simulink model "NL_Simulation"  (R2018b)
settings: Solver=VariableStepAuto  StartTime=0.0  StopTime=.5  FixedStep=0.01
values from neighbouring files (symbols this model uses):
  StateVals = SetInitial(Vinf,AeroType)    [setup_NL.m]
undefined symbols (not defined in the file or in its folder): AC
libraries: Tools_6dofSimulation x12, aerolibatmos2 x1, shared6dof x1, aerolibasang x1, dspmathops x1
settings Model: Creator=abhineet  LastModifiedBy=abhineet
settings DataIOCC: ExternalInput=getinputstruct(op_trim1)  InitialState=getstatestruct(op_trim1)  SaveOutput=off  SignalLogging=off  DSMLogging=off  SaveTime=off
settings DebuggingCC: ReadBeforeWriteMsg=DisableAll  WriteAfterWriteMsg=DisableAll  WriteAfterReadMsg=DisableAll  MultiTaskDSMMsg=none  SignalLabelMismatchMsg=warning  LibraryContextMissingDiagnostic=none  StrictBusMsg=ErrorOnBusTreatedAsVector  NonBusSignalsTreatedAsBus=warning
settings ModelReferenceCC: UpdateModelReferenceTargets=IfOutOfDate
settings SFSimCC: SFSimEcho=off  SimUseLocalCustomCode=off
settings RTWCC: RTWUseLocalCustomCode=off

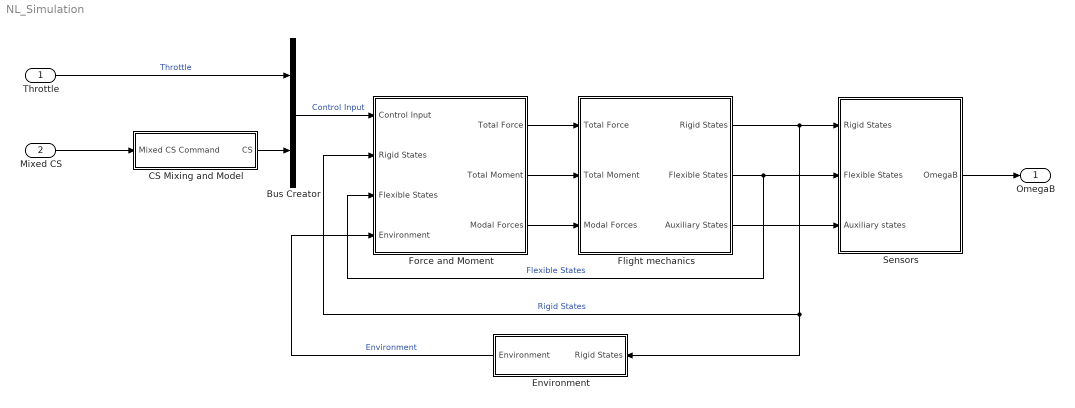
== system NL_Simulation ==
  Throttle : Inport
  Mixed CS : Inport  Port=2
  Bus Creator : BusCreator  Inputs=2
  CS Mixing and Model : Subsystem
  Environment : Subsystem
  Flight mechanics : Subsystem
  "Force and Moment " : Subsystem
  Sensors : Subsystem
  OmegaB : Outport
  wires:
  "Force and Moment "/1(Total Force) -> Flight mechanics/1(Total Force)
  "Force and Moment "/2(Total Moment) -> Flight mechanics/2(Total Moment)
  Bus Creator/1 -> "Force and Moment "/1(Control Input)  "Control Input"
  Flight mechanics/1(Rigid States) -> Sensors/1(Rigid States), "Force and Moment "/2(Rigid States), Environment/1(Rigid States)  "Rigid States"
  "Force and Moment "/3(Modal Forces) -> Flight mechanics/3(Modal Forces)
  Flight mechanics/2(Flexible States) -> Sensors/2(Flexible States), "Force and Moment "/3(Flexible States)  "Flexible States"
  Flight mechanics/3(Auxiliary States) -> Sensors/3(Auxiliary states)
  Environment/1(Environment) -> "Force and Moment "/4(Environment)  "Environment"
  CS Mixing and Model/1(CS) -> Bus Creator/2
  Throttle/1 -> Bus Creator/1  "Throttle"
  Mixed CS/1 -> CS Mixing and Model/1(Mixed CS Command)
  Sensors/1(OmegaB) -> OmegaB/1

== system NL_Simulation/CS Mixing and Model ==
  Mixed CS Command : Inport
  CS Mixing : Subsystem
  CS Model : Subsystem
  CS : Outport
  wires:
  CS Mixing/1(CS Command) -> CS Model/1(CS Command)
  Mixed CS Command/1 -> CS Mixing/1(Mixed CS Command)
  CS Model/1(CS) -> CS/1

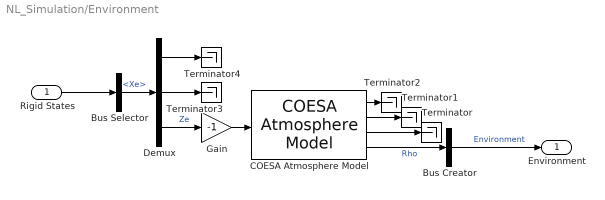
== system NL_Simulation/Environment ==
  Rigid States : Inport
  Bus Creator : BusCreator  Inputs=1
  Bus Selector : BusSelector  OutputSignals=Xe
  COESA Atmosphere Model : aerolibatmos2/COESA Atmosphere Model  units=Metric (MKS)  spec=1976 COESA-extended U.S. Standard Atmosphere  model=Profile  profile_var=High temperature  profile_percent=1%  profile_alt=5 km (16404 ft)  envelope_var=High temperature  envelope_percent=1%  action=Warning
  Demux : Demux  Outputs=3
  Gain : Gain  Gain=-1
  Terminator{,1..4} (5 alike) : Terminator
  Environment : Outport
  wires:
  Rigid States/1 -> Bus Selector/1
  COESA Atmosphere Model/1 -> Terminator2/1
  COESA Atmosphere Model/2 -> Terminator1/1
  COESA Atmosphere Model/3 -> Terminator/1
  COESA Atmosphere Model/4 -> Bus Creator/1  "Rho"
  Bus Creator/1 -> Environment/1  "Environment"
  Bus Selector/1 -> Demux/1  "<Xe>"
  Demux/2 -> Terminator3/1
  Demux/1 -> Terminator4/1
  Demux/3 -> Gain/1  "Ze"
  Gain/1 -> COESA Atmosphere Model/1

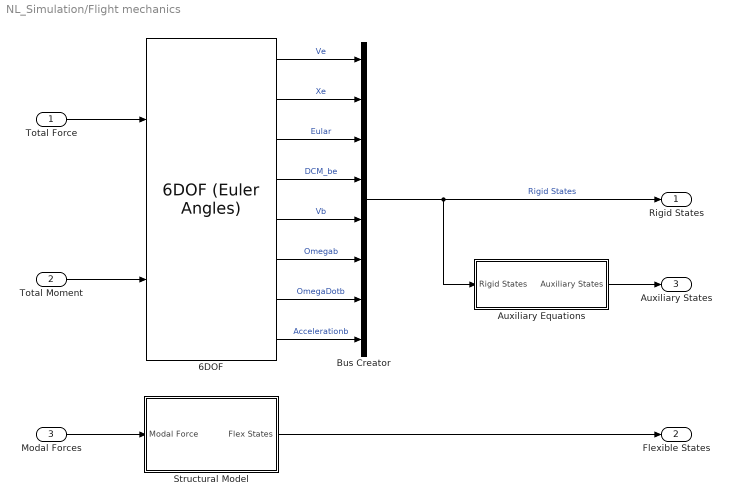
== system NL_Simulation/Flight mechanics ==
  Total Force : Inport
  Total Moment : Inport  Port=2
  Modal Forces : Inport  Port=3
  6DOF : shared6dof/6DOF (Euler Angles)  units=Metric (MKS)  mtype=Fixed  rep=Euler Angles  xme_0=StateVals.Xe  Vm_0=StateVals.Vb  eul_0=StateVals.Eular  pm_0=StateVals.AngRates  mass_0=AC.MassProp.mass  mass_e=0.5  mass_f=2.0  inertia=AC.MassProp.inertia  inertia_e=eye(3)  inertia_f=2*eye(3)  k_quat=1.0  vre_flag=on  abi_flag=off  aMode=0  xme_statename=''  Vm_statename=''  eul_statename=''  quat_statename=''  pm_statename=''  mass_statename=''
      settings: SourceProductBaseCode=AE
  "Auxiliary Equations " : Subsystem
  Bus Creator : BusCreator  Inputs=8
  Structural Model : Subsystem
  Rigid States : Outport
  Flexible States : Outport  Port=2
  Auxiliary States : Outport  Port=3
  wires:
  6DOF/8 -> Bus Creator/8  "Accelerationb"
  6DOF/6 -> Bus Creator/6  "Omegab"
  6DOF/1 -> Bus Creator/1  "Ve"
  6DOF/7 -> Bus Creator/7  "OmegaDotb"
  Total Moment/1 -> 6DOF/2
  6DOF/2 -> Bus Creator/2  "Xe"
  6DOF/4 -> Bus Creator/4  "DCM_be"
  6DOF/3 -> Bus Creator/3  "Eular"
  Total Force/1 -> 6DOF/1
  6DOF/5 -> Bus Creator/5  "Vb"
  "Auxiliary Equations "/1(Auxiliary States) -> Auxiliary States/1
  Bus Creator/1 -> Rigid States/1, "Auxiliary Equations "/1(Rigid States)  "Rigid States"
  Structural Model/1(Flex States) -> Flexible States/1
  Modal Forces/1 -> Structural Model/1(Modal Force)

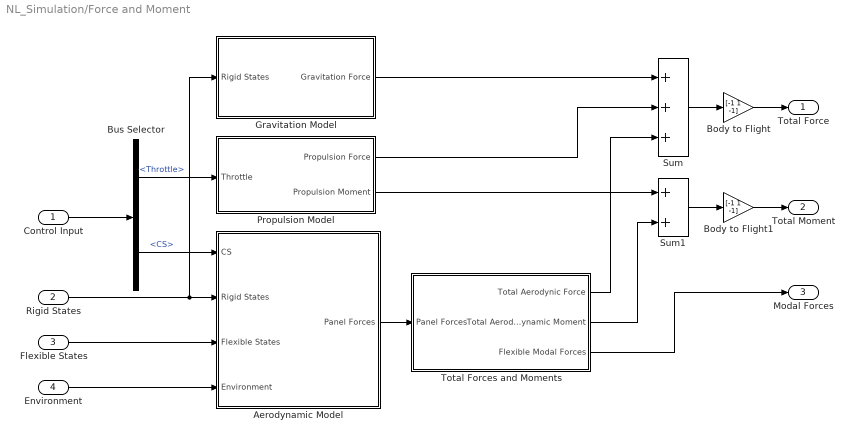
== system NL_Simulation/Force and Moment  ==
  Control Input : Inport
  Rigid States : Inport  Port=2
  Flexible States : Inport  Port=3
  Environment : Inport  Port=4
  Aerodynamic Model : Subsystem
  Body to Flight : Gain  Gain=[-1 1 -1]
  Body to Flight1 : Gain  Gain=[-1 1 -1]
  Bus Selector : BusSelector  OutputSignals=Throttle,CS
  Gravitation Model : Subsystem
  Propulsion Model : Subsystem
  Sum : Sum  Inputs=+++
  Sum1 : Sum
  Total Forces and Moments : Subsystem
  Total Force : Outport
  Total Moment : Outport  Port=2
  Modal Forces : Outport  Port=3
  wires:
  Control Input/1 -> Bus Selector/1
  Bus Selector/1 -> Propulsion Model/1(Throttle)  "<Throttle>"
  Bus Selector/2 -> Aerodynamic Model/1(CS)  "<CS>"
  Rigid States/1 -> Gravitation Model/1(Rigid States), Aerodynamic Model/2(Rigid States)
  Flexible States/1 -> Aerodynamic Model/3(" Flexible States")
  Sum/1 -> Body to Flight/1
  Environment/1 -> Aerodynamic Model/4(Environment)
  Total Forces and Moments/3(Flexible Modal Forces) -> Modal Forces/1
  Total Forces and Moments/1(Total Aerodynic Force) -> Sum/3
  Total Forces and Moments/2(Total Aerodynamic Moment) -> Sum1/2
  Aerodynamic Model/1(Panel Forces) -> Total Forces and Moments/1(Panel Forces)
  Propulsion Model/1(Propulsion Force) -> Sum/2
  Gravitation Model/1(Gravitation Force) -> Sum/1
  Propulsion Model/2(Propulsion Moment) -> Sum1/1
  Sum1/1 -> Body to Flight1/1
  Body to Flight/1 -> Total Force/1
  Body to Flight1/1 -> Total Moment/1

== system NL_Simulation/Sensors ==
  Rigid States : Inport
  Flexible States : Inport  Port=2
  Auxiliary states : Inport  Port=3
  Bus Selector : BusSelector  OutputSignals=Omegab
  Terminator1 : Terminator
  Terminator2 : Terminator
  OmegaB : Outport
  wires:
  Rigid States/1 -> Bus Selector/1
  Flexible States/1 -> Terminator1/1
  Auxiliary states/1 -> Terminator2/1
  Bus Selector/1 -> OmegaB/1  "<Omegab>"

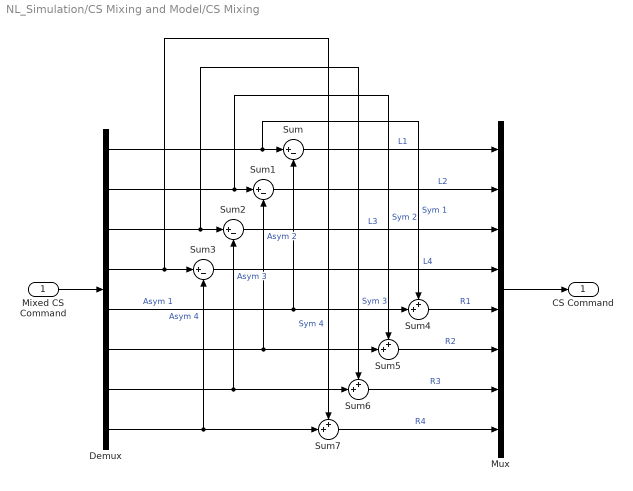
== system NL_Simulation/CS Mixing and Model/CS Mixing ==
  Mixed CS Command : Inport
  Demux : Demux  Outputs=8
  Mux : Mux  Inputs=8
  Sum{,1..3} (4 alike) : Sum  Inputs=|+-
  Sum{4..7} (4 alike) : Sum  Inputs=++|
  CS Command : Outport
  wires:
  Demux/7 -> Sum6/2, Sum2/2  "Asym 3"
  Sum/1 -> Mux/1  "L1"
  Sum4/1 -> Mux/5  "R1"
  Sum7/1 -> Mux/8  "R4"
  Demux/8 -> Sum7/2, Sum3/2  "Asym 4"
  Demux/2 -> Sum5/1, Sum1/1  "Sym 2"
  Demux/1 -> Sum4/1, Sum/1  "Sym 1"
  Demux/4 -> Sum7/1, Sum3/1  "Sym 4"
  Sum1/1 -> Mux/2  "L2"
  Demux/5 -> Sum4/2, Sum/2  "Asym 1"
  Sum2/1 -> Mux/3  "L3"
  Demux/3 -> Sum6/1, Sum2/1  "Sym 3"
  Sum5/1 -> Mux/6  "R2"
  Sum6/1 -> Mux/7  "R3"
  Demux/6 -> Sum5/2, Sum1/2  "Asym 2"
  Mixed CS Command/1 -> Demux/1
  Sum3/1 -> Mux/4  "L4"
  Mux/1 -> CS Command/1

== system NL_Simulation/CS Mixing and Model/CS Model ==
  CS Command : Inport
  Bus Creator : BusCreator  Inputs=2
  CS Pos : Integrator  InitialCondition=StateVals.CSPos
  Gain : Gain  Gain=AC.CS.CSTau
  Sum : Sum  Inputs=|+-
  CS : Outport
  wires:
  CS Command/1 -> Sum/1
  Sum/1 -> Gain/1
  Gain/1 -> Bus Creator/2, CS Pos/1  "CS Vel"
  CS Pos/1 -> Bus Creator/1, Sum/2  "CS Pos"
  Bus Creator/1 -> CS/1  "CS"

== system NL_Simulation/Flight mechanics/Auxiliary Equations  ==
  Rigid States : Inport
  Bus Creator1 : BusCreator  Inputs=3
  Bus Selector : BusSelector  OutputSignals=Vb
  "Incidence, Sideslip, & Airspeed" : aerolibasang/Incidence, Sideslip, & Airspeed
      settings: SourceProductName=Aerospace Blockset
  Auxiliary States : Outport
  wires:
  Bus Creator1/1 -> Auxiliary States/1  "Wind Parameters"
  "Incidence, Sideslip, & Airspeed"/3 -> Bus Creator1/3  "vinf"
  "Incidence, Sideslip, & Airspeed"/2 -> Bus Creator1/2  "beta"
  "Incidence, Sideslip, & Airspeed"/1 -> Bus Creator1/1  "alpha"
  Rigid States/1 -> Bus Selector/1  "Rigid States"
  Bus Selector/1 -> "Incidence, Sideslip, & Airspeed"/1  "<Vb>"

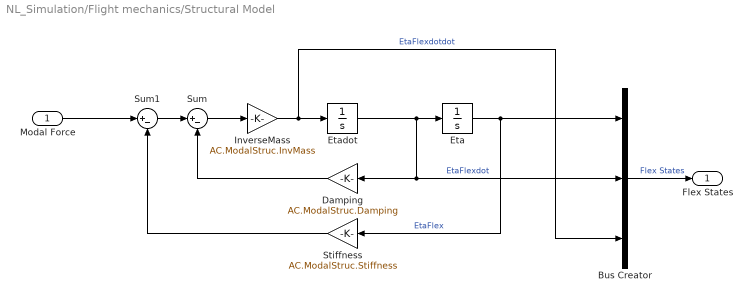
== system NL_Simulation/Flight mechanics/Structural Model ==
  Modal Force : Inport
  Bus Creator : BusCreator  Inputs=3
  Damping : Gain  Gain=AC.ModalStruc.Damping
  Eta : Integrator  InitialCondition=StateVals.Eta
  Etadot : Integrator  InitialCondition=StateVals.EtaDot
  InverseMass : Gain  Gain=AC.ModalStruc.InvMass
  Stiffness : Gain  Gain=AC.ModalStruc.Stiffness
  Sum : Sum  Inputs=|+-
  Sum1 : Sum  Inputs=|+-
  Flex States : Outport
  wires:
  InverseMass/1 -> Bus Creator/3, Etadot/1  "EtaFlexdotdot"
  Etadot/1 -> Damping/1, Bus Creator/2, Eta/1  "EtaFlexdot"
  Damping/1 -> Sum/2
  Eta/1 -> Bus Creator/1, Stiffness/1  "EtaFlex"
  Sum/1 -> InverseMass/1
  Sum1/1 -> Sum/1
  Modal Force/1 -> Sum1/1
  Bus Creator/1 -> Flex States/1  "Flex States"
  Stiffness/1 -> Sum1/2

== system NL_Simulation/Force and Moment /Aerodynamic Model ==
  CS : Inport
  Rigid States : Inport  Port=2
  " Flexible States" : Inport  Port=3
  Environment : Inport  Port=4
  Steady Aerodynamics : Subsystem
  Sum : Sum
  Unsteady Aerodynamics : Subsystem
  Panel Forces : Outport
  wires:
  CS/1 -> Steady Aerodynamics/1(CS)
  Rigid States/1 -> Unsteady Aerodynamics/1(Rigid States), Steady Aerodynamics/2(Rigid States)
  " Flexible States"/1 -> Unsteady Aerodynamics/2(Flexible States), Steady Aerodynamics/3(Flexible States)
  Environment/1 -> Steady Aerodynamics/4(Environment)
  Steady Aerodynamics/1(Total Steady Forces) -> Sum/1
  Sum/1 -> Panel Forces/1
  Unsteady Aerodynamics/1(Total Unsteady Forces) -> Sum/2

== system NL_Simulation/Force and Moment /Gravitation Model ==
  Rigid States : Inport
  Bus Selector : BusSelector  OutputSignals=DCM_be
  Flight to Body Axes : Gain  Gain=[-1 1 -1]
  Mass : Constant  Value=AC.MassProp.mass
  Product1 : Product
  Product2 : Product  Multiplication=Matrix(*)
  Selector : Selector  NumberOfDimensions=2  InputPortWidth=3  IndexOptions=Select all,Index vector (dialog)  Indices=[1 3],3  OutputSizes=1,1
  g : Constant  Value=9.81
  Gravitation Force : Outport
  wires:
  Rigid States/1 -> Bus Selector/1
  Bus Selector/1 -> Selector/1  "<DCM_be>"
  Mass/1 -> Product1/2
  g/1 -> Product1/1
  Product1/1 -> Product2/2  "mg"
  Flight to Body Axes/1 -> Gravitation Force/1
  Selector/1 -> Product2/1
  Product2/1 -> Flight to Body Axes/1

== system NL_Simulation/Force and Moment /Propulsion Model ==
  Throttle : Inport
  Gain : Gain  Gain=[-100 0 0]
  Gain1 : Gain  Gain=[0 0 0]
  Propulsion Force : Outport
  Propulsion Moment : Outport  Port=2
  wires:
  Gain/1 -> Propulsion Force/1
  Throttle/1 -> Gain1/1, Gain/1
  Gain1/1 -> Propulsion Moment/1

== system NL_Simulation/Force and Moment /Total Forces and Moments ==
  Panel Forces : Inport
  Constant1 : Constant  Value=AC.Aero.VLMData.grid.r_cgvortex
  MATLAB Function : MATLAB Function  TreatAsAtomicUnit=on
  RB Mode Tranlation : Gain  Gain=AC.ModalStruc.Phif_aero_trans'  Multiplication=Matrix(K*u)
  Reshape : Reshape
  Reshape1 : Reshape
  Sum : Sum  Inputs=+  CollapseMode=Specified dimension  CollapseDim=2
  Total Aerodynic Force : Outport
  Total Aerodynamic Moment : Outport  Port=2
  Flexible Modal Forces : Outport  Port=3
  wires:
  MATLAB Function/1(SumRcrossF) -> Total Aerodynamic Moment/1
  RB Mode Tranlation/1 -> Flexible Modal Forces/1
  Reshape/1 -> RB Mode Tranlation/1
  Panel Forces/1 -> Reshape/1, MATLAB Function/2(F), Sum/1
  Constant1/1 -> MATLAB Function/1(R)
  Sum/1 -> Reshape1/1
  Reshape1/1 -> Total Aerodynic Force/1

== system NL_Simulation/Force and Moment /Aerodynamic Model/Steady Aerodynamics ==
  CS : Inport
  Rigid States : Inport  Port=2
  Flexible States : Inport  Port=3
  Environment : Inport  Port=4
  N_hat : Subsystem
  Normal Wash : Subsystem
  Panel Forces Calculation : Subsystem
  Total Wash : Subsystem
  Vortex Strength : Subsystem
  Total Steady Forces : Outport
  wires:
  N_hat/1(Nhat) -> Normal Wash/1(Nhat)
  Normal Wash/1(Normal Wash) -> Vortex Strength/2(External Normalwash)
  Total Wash/1(Total Wash) -> Normal Wash/2(Total Wash)
  Panel Forces Calculation/1(Panel Forces) -> Total Steady Forces/1
  Rigid States/1 -> Panel Forces Calculation/1(Rigid States), Total Wash/1(Rigid States)
  Vortex Strength/1(Gamma) -> Panel Forces Calculation/3(Gamma)
  Environment/1 -> Panel Forces Calculation/4(Environment)
  CS/1 -> N_hat/1(CS)
  Flexible States/1 -> Vortex Strength/1(Flexible States), Panel Forces Calculation/2(Flexible States), N_hat/2(Flexible States), Total Wash/2(Flexible States)

== system NL_Simulation/Force and Moment /Aerodynamic Model/Unsteady Aerodynamics ==
  Rigid States : Inport
  Flexible States : Inport  Port=2
  MATLAB Function : MATLAB Function  TreatAsAtomicUnit=on
  Nhat0 : Constant  Value=AC.Aero.Nhat0
  Normal Forces : Subsystem
  Normal Wash Derivative : Subsystem
  Total Wash Derivative : Subsystem
      mask init:
      | %% All modes
      | Sys_Ab = ss(-300,1,1,0)*eye(3);
      | Sys_OmegaDotb = ss(-300,1,1,0)*eye(3);
      | Sys_FlexDotDotb = ss(-300,1,1,0)*eye(6);
  Total Unsteady Forces : Outport
  wires:
  Rigid States/1 -> Total Wash Derivative/1(Rigid States), Normal Forces/2(Rigid States)
  Flexible States/1 -> Total Wash Derivative/2(Flexible States)
  Normal Wash Derivative/1(Normal Wash Derivative) -> Normal Forces/1(Normal Wash Derivatives)
  Nhat0/1 -> MATLAB Function/1(nhat0)
  Normal Forces/1(Normal Forces) -> MATLAB Function/2(NormalForces)
  MATLAB Function/1(TotalForces) -> Total Unsteady Forces/1
  Total Wash Derivative/1(Total Wash Derivatives) -> Normal Wash Derivative/1(Total Wash Derivative)

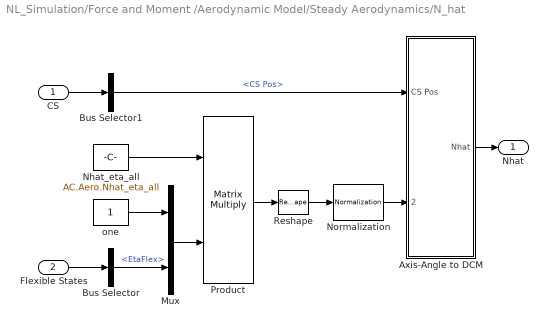
== system NL_Simulation/Force and Moment /Aerodynamic Model/Steady Aerodynamics/N_hat ==
  CS : Inport
  Flexible States : Inport  Port=2
  Axis-Angle to DCM : Subsystem
  Bus Selector : BusSelector  OutputSignals=EtaFlex
  Bus Selector1 : BusSelector  OutputSignals=CS Pos
  Mux : Mux  Inputs=2
  Nhat_eta_all : Constant  Value=AC.Aero.Nhat_eta_all
  Normalization : dspmathops/Normalization  NormType=2-norm  Bias=1e-10  NormOver=Each column  Dimension=1  roundingMode=Floor  overflowMode=off  accumDataTypeStr=Inherit: Same as product output  accumLastDataTypeStr=Inherit: Same as product output  outputDataTypeStr=Inherit: Same as product output  outputMin=[]  outputMax=[]  outputLastDataTypeStr=Inherit: Same as product output
      settings: SourceProductName=DSP System Toolbox
  Product : Product  Multiplication=Matrix(*)
  Reshape : Reshape  OutputDimensionality=Customize  OutputDimensions=[3,AC.Aero.NumPanels]
  one : Constant
  Nhat : Outport
  wires:
  Flexible States/1 -> Bus Selector/1
  Product/1 -> Reshape/1
  Nhat_eta_all/1 -> Product/1
  CS/1 -> Bus Selector1/1
  Bus Selector1/1 -> Axis-Angle to DCM/1(CS Pos)  "<CS Pos>"
  Axis-Angle to DCM/1(Nhat) -> Nhat/1
  Reshape/1 -> Normalization/1
  Normalization/1 -> Axis-Angle to DCM/2(Nhat_Flex)
  Bus Selector/1 -> Mux/2  "<EtaFlex>"
  one/1 -> Mux/1
  Mux/1 -> Product/2

== system NL_Simulation/Force and Moment /Aerodynamic Model/Steady Aerodynamics/Normal Wash ==
  Nhat : Inport
  Total Wash : Inport  Port=2
  Product : Product
  Sum : Sum  Inputs=+  CollapseMode=Specified dimension
  Transpose : Math  Operator=transpose  SaturateOnIntegerOverflow=on
  Normal Wash : Outport
  wires:
  Nhat/1 -> Product/1
  Total Wash/1 -> Product/2
  Product/1 -> Sum/1
  Sum/1 -> Transpose/1
  Transpose/1 -> Normal Wash/1

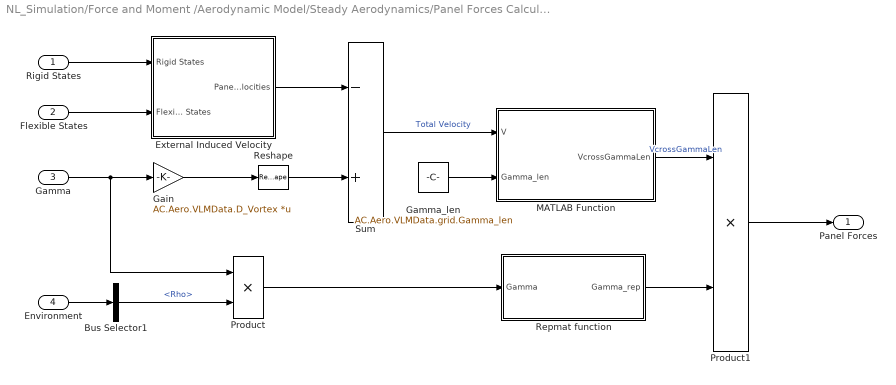
== system NL_Simulation/Force and Moment /Aerodynamic Model/Steady Aerodynamics/Panel Forces Calculation ==
  Rigid States : Inport
  Flexible States : Inport  Port=2
  Gamma : Inport  Port=3
  Environment : Inport  Port=4
  Bus Selector1 : BusSelector  OutputSignals=Rho
  External Induced Velocity : Subsystem
  Gain : Gain  Gain=AC.Aero.VLMData.D_Vortex  Multiplication=Matrix(K*u)
  Gamma_len : Constant  Value=AC.Aero.VLMData.grid.Gamma_len
  MATLAB Function : MATLAB Function  TreatAsAtomicUnit=on
  Product : Product
  Product1 : Product
  Repmat function : MATLAB Function  TreatAsAtomicUnit=on
  Reshape : Reshape  OutputDimensionality=Customize  OutputDimensions=[3,AC.Aero.NumPanels]
  Sum : Sum  Inputs=-+
  Panel Forces : Outport
  wires:
  Rigid States/1 -> External Induced Velocity/1(Rigid States)
  Flexible States/1 -> External Induced Velocity/2(Flexible States)
  External Induced Velocity/1(Panel Velocities) -> Sum/1
  Environment/1 -> Bus Selector1/1
  Gain/1 -> Reshape/1
  Reshape/1 -> Sum/2
  Gamma/1 -> Product/1, Gain/1
  Sum/1 -> MATLAB Function/1(V)  "Total Velocity"
  Gamma_len/1 -> MATLAB Function/2(Gamma_len)
  Bus Selector1/1 -> Product/2  "<Rho>"
  Product/1 -> Repmat function/1(Gamma)
  Repmat function/1(Gamma_rep) -> Product1/2
  Product1/1 -> Panel Forces/1
  MATLAB Function/1(VcrossGammaLen) -> Product1/1  "VcrossGammaLen"

== system NL_Simulation/Force and Moment /Aerodynamic Model/Steady Aerodynamics/Total Wash ==
  Rigid States : Inport
  Flexible States : Inport  Port=2
  Bus Selector : BusSelector  OutputSignals=Vb,Omegab
  Flexible defections : Subsystem
  Gain : Gain  Gain=[-1,1,-1]
  Gain1 : Gain  Gain=[-1,1,-1]
  Repmat function : MATLAB Function  TreatAsAtomicUnit=on  mask{NumPanels=AC.Aero.NumPanels}
      mask prompts: NumPanels "Number of Panels"
      mask init:
      | % NumPanels = 888;
  Sum : Sum  Inputs=+++
  Vel_Omega : Subsystem
  Total Wash : Outport
  wires:
  Rigid States/1 -> Bus Selector/1
  Bus Selector/1 -> Gain/1  "<Vb>"
  Bus Selector/2 -> Gain1/1  "<Omegab>"
  Vel_Omega/1(Omegacrossr) -> Sum/2
  Gain/1 -> Repmat function/1(V)
  Gain1/1 -> Vel_Omega/1(Omegab)
  Flexible States/1 -> Flexible defections/1(Flexible States)
  Flexible defections/1(Del_r_flex) -> Vel_Omega/2(Del_r_flex)
  Flexible defections/2(Del_v_flex) -> Sum/3
  Sum/1 -> Total Wash/1
  Repmat function/1(Vrepmat) -> Sum/1

== system NL_Simulation/Force and Moment /Aerodynamic Model/Steady Aerodynamics/Vortex Strength ==
  Flexible States : Inport
  External Normalwash : Inport  Port=2
  Product : Product  Multiplication=Matrix(*)
  Subsystem : Subsystem
  Gamma : Outport
  wires:
  External Normalwash/1 -> Product/2
  Product/1 -> Gamma/1
  Flexible States/1 -> Subsystem/1(Flexible States)
  Subsystem/1(AIC) -> Product/1

== system NL_Simulation/Force and Moment /Aerodynamic Model/Unsteady Aerodynamics/Normal Forces ==
  Normal Wash Derivatives : Inport
  Rigid States : Inport  Port=2
  Gain : Gain  Gain=AC.Aero.DLMData.A1  Multiplication=Matrix(K*u)
  Gain1 : Gain  Gain=AC.Aero.DLMData.Clag  Multiplication=Matrix(K*u)
  MACby2V : Subsystem
  Product : Product
  Subsystem1 : Subsystem
  Sum : Sum
  Normal Forces : Outport
  wires:
  Normal Wash Derivatives/1 -> Product/1, Subsystem1/1(Normal Wash Derivative)
  Sum/1 -> Normal Forces/1
  Rigid States/1 -> MACby2V/1(Rigid States)
  MACby2V/1(MACby2V) -> Subsystem1/2(b_over_V), Product/2
  Product/1 -> Gain/1
  Gain/1 -> Sum/1
  Subsystem1/1(Lag States) -> Gain1/1
  Gain1/1 -> Sum/2

== system NL_Simulation/Force and Moment /Aerodynamic Model/Unsteady Aerodynamics/Normal Wash Derivative ==
  Total Wash Derivative : Inport
  Constant : Constant  Value=AC.Aero.Nhat0
  Product : Product
  Sum : Sum  Inputs=+  CollapseMode=Specified dimension
  Transpose : Math  Operator=transpose  SaturateOnIntegerOverflow=on
  Normal Wash Derivative : Outport
  wires:
  Sum/1 -> Transpose/1
  Constant/1 -> Product/1
  Total Wash Derivative/1 -> Product/2
  Product/1 -> Sum/1
  Transpose/1 -> Normal Wash Derivative/1

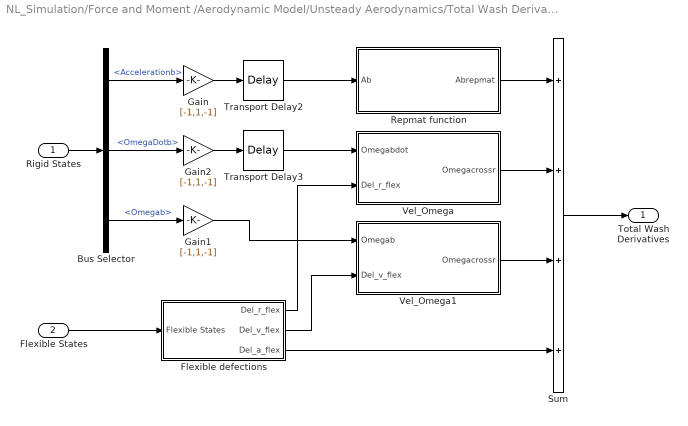
== system NL_Simulation/Force and Moment /Aerodynamic Model/Unsteady Aerodynamics/Total Wash Derivative ==
  Rigid States : Inport
  Flexible States : Inport  Port=2
  Bus Selector : BusSelector  OutputSignals=Accelerationb,OmegaDotb,Omegab
  Flexible defections : Subsystem
  Gain : Gain  Gain=[-1,1,-1]
  Gain1 : Gain  Gain=[-1,1,-1]
  Gain2 : Gain  Gain=[-1,1,-1]
  Repmat function : MATLAB Function  TreatAsAtomicUnit=on  mask{NumPanels=AC.Aero.NumPanels}
      mask prompts: NumPanels "Number of Panels"
      mask init:
      | % NumPanels = 888;
  Sum : Sum  Inputs=++++
  Transport Delay2 : TransportDelay  DelayTime=0.001
  Transport Delay3 : TransportDelay  DelayTime=0.001
  Vel_Omega : Subsystem
  Vel_Omega1 : Subsystem
  Total Wash Derivatives : Outport
  wires:
  Rigid States/1 -> Bus Selector/1
  Bus Selector/1 -> Gain/1  "<Accelerationb>"
  Vel_Omega/1(Omegacrossr) -> Sum/2
  Gain2/1 -> Transport Delay3/1
  Flexible States/1 -> Flexible defections/1(Flexible States)
  Sum/1 -> Total Wash Derivatives/1
  Repmat function/1(Abrepmat) -> Sum/1
  Bus Selector/2 -> Gain2/1  "<OmegaDotb>"
  Flexible defections/2(Del_v_flex) -> Vel_Omega1/2(Del_v_flex)
  Vel_Omega1/1(Omegacrossr) -> Sum/3
  Flexible defections/1(Del_r_flex) -> Vel_Omega/2(Del_r_flex)
  Gain/1 -> Transport Delay2/1
  Flexible defections/3(Del_a_flex) -> Sum/4
  Bus Selector/3 -> Gain1/1  "<Omegab>"
  Gain1/1 -> Vel_Omega1/1(Omegab)
  Transport Delay2/1 -> Repmat function/1(Ab)
  Transport Delay3/1 -> Vel_Omega/1(Omegabdot)

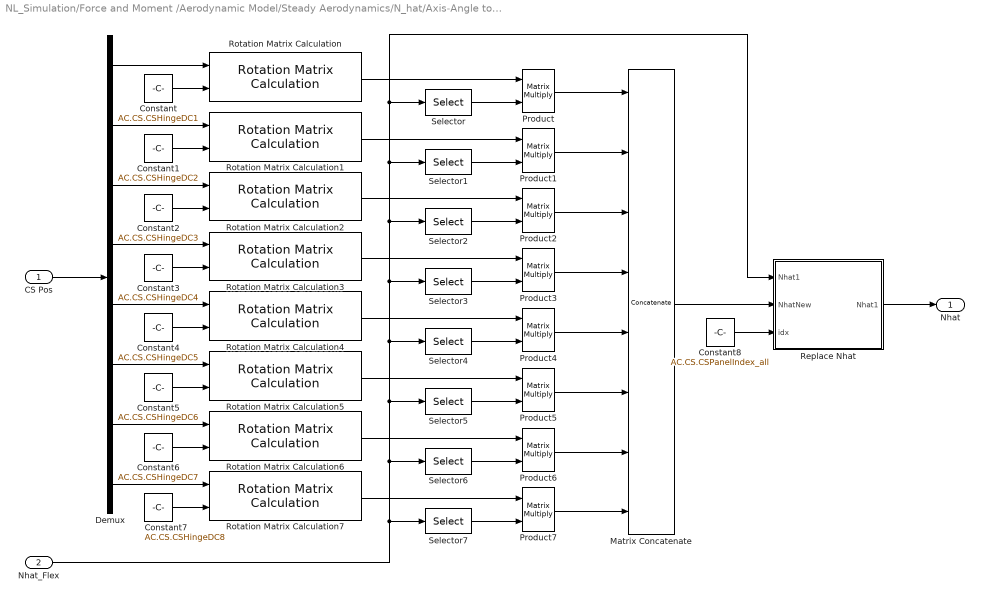
== system NL_Simulation/Force and Moment /Aerodynamic Model/Steady Aerodynamics/N_hat/Axis-Angle to DCM ==
  CS Pos : Inport
  Nhat_Flex : Inport  Port=2
  Constant : Constant  Value=AC.CS.CSHingeDC1
  Constant1 : Constant  Value=AC.CS.CSHingeDC2
  Constant2 : Constant  Value=AC.CS.CSHingeDC3
  Constant3 : Constant  Value=AC.CS.CSHingeDC4
  Constant4 : Constant  Value=AC.CS.CSHingeDC5
  Constant5 : Constant  Value=AC.CS.CSHingeDC6
  Constant6 : Constant  Value=AC.CS.CSHingeDC7
  Constant7 : Constant  Value=AC.CS.CSHingeDC8
  Constant8 : Constant  Value=AC.CS.CSPanelIndex_all
  Demux : Demux  Outputs=8
  Matrix Concatenate : Concatenate  NumInputs=8  Mode=Multidimensional array  ConcatenateDimension=2
  Product{,1..7} (8 alike) : Product  Multiplication=Matrix(*)
  Replace Nhat : MATLAB Function  TreatAsAtomicUnit=on
  Rotation Matrix Calculation{,1..7} (8 alike) : Tools_6dofSimulation/Rotation Matrix Calculation  SystemSampleTime=-1
  Selector : Selector  NumberOfDimensions=2  InputPortWidth=3  IndexOptions=Select all,Index vector (dialog)  Indices=[1 3],AC.CS.CSPanelIndex1  OutputSizes=1,1
  Selector1 : Selector  NumberOfDimensions=2  InputPortWidth=3  IndexOptions=Select all,Index vector (dialog)  Indices=[1 3],AC.CS.CSPanelIndex2  OutputSizes=1,1
  Selector2 : Selector  NumberOfDimensions=2  InputPortWidth=3  IndexOptions=Select all,Index vector (dialog)  Indices=[1 3],AC.CS.CSPanelIndex3  OutputSizes=1,1
  Selector3 : Selector  NumberOfDimensions=2  InputPortWidth=3  IndexOptions=Select all,Index vector (dialog)  Indices=[1 3],AC.CS.CSPanelIndex4  OutputSizes=1,1
  Selector4 : Selector  NumberOfDimensions=2  InputPortWidth=3  IndexOptions=Select all,Index vector (dialog)  Indices=[1 3],AC.CS.CSPanelIndex5  OutputSizes=1,1
  Selector5 : Selector  NumberOfDimensions=2  InputPortWidth=3  IndexOptions=Select all,Index vector (dialog)  Indices=[1 3],AC.CS.CSPanelIndex6  OutputSizes=1,1
  Selector6 : Selector  NumberOfDimensions=2  InputPortWidth=3  IndexOptions=Select all,Index vector (dialog)  Indices=[1 3],AC.CS.CSPanelIndex7  OutputSizes=1,1
  Selector7 : Selector  NumberOfDimensions=2  InputPortWidth=3  IndexOptions=Select all,Index vector (dialog)  Indices=[1 3],AC.CS.CSPanelIndex8  OutputSizes=1,1
  Nhat : Outport
  wires:
  CS Pos/1 -> Demux/1
  Demux/1 -> Rotation Matrix Calculation/1
  Demux/2 -> Rotation Matrix Calculation1/1
  Demux/3 -> Rotation Matrix Calculation2/1
  Demux/4 -> Rotation Matrix Calculation3/1
  Demux/5 -> Rotation Matrix Calculation4/1
  Demux/6 -> Rotation Matrix Calculation5/1
  Demux/7 -> Rotation Matrix Calculation6/1
  Demux/8 -> Rotation Matrix Calculation7/1
  Constant/1 -> Rotation Matrix Calculation/2
  Constant1/1 -> Rotation Matrix Calculation1/2
  Constant2/1 -> Rotation Matrix Calculation2/2
  Constant3/1 -> Rotation Matrix Calculation3/2
  Constant4/1 -> Rotation Matrix Calculation4/2
  Constant5/1 -> Rotation Matrix Calculation5/2
  Constant6/1 -> Rotation Matrix Calculation6/2
  Constant7/1 -> Rotation Matrix Calculation7/2
  Rotation Matrix Calculation/1 -> Product/1
  Rotation Matrix Calculation1/1 -> Product1/1
  Rotation Matrix Calculation2/1 -> Product2/1
  Rotation Matrix Calculation3/1 -> Product3/1
  Rotation Matrix Calculation4/1 -> Product4/1
  Rotation Matrix Calculation6/1 -> Product6/1
  Rotation Matrix Calculation7/1 -> Product7/1
  Nhat_Flex/1 -> Replace Nhat/1("Nhat1 "), Selector/1, Selector1/1, Selector2/1, Selector3/1, Selector4/1, Selector5/1, Selector6/1, Selector7/1
  Selector/1 -> Product/2
  Selector1/1 -> Product1/2
  Selector2/1 -> Product2/2
  Selector3/1 -> Product3/2
  Selector4/1 -> Product4/2
  Rotation Matrix Calculation5/1 -> Product5/1
  Selector5/1 -> Product5/2
  Selector6/1 -> Product6/2
  Selector7/1 -> Product7/2
  Constant8/1 -> Replace Nhat/3(idx)
  Product1/1 -> Matrix Concatenate/2
  Product2/1 -> Matrix Concatenate/3
  Product3/1 -> Matrix Concatenate/4
  Product4/1 -> Matrix Concatenate/5
  Product5/1 -> Matrix Concatenate/6
  Product6/1 -> Matrix Concatenate/7
  Product7/1 -> Matrix Concatenate/8
  Replace Nhat/1(Nhat1) -> Nhat/1
  Product/1 -> Matrix Concatenate/1
  Matrix Concatenate/1 -> Replace Nhat/2(NhatNew)

== system NL_Simulation/Force and Moment /Aerodynamic Model/Steady Aerodynamics/Panel Forces Calculation/External Induced Velocity ==
  Rigid States : Inport
  Flexible States : Inport  Port=2
  Bus Selector : BusSelector  OutputSignals=Vb,Omegab
  Flexible defections : Subsystem
  Gain : Gain  Gain=[-1,1,-1]
  Gain1 : Gain  Gain=[-1,1,-1]
  Repmat function : MATLAB Function  TreatAsAtomicUnit=on  mask{NumPanels=AC.Aero.NumPanels}
      mask prompts: NumPanels "Number of Panels"
      mask init:
      | % NumPanels = 888;
  Sum : Sum  Inputs=+++
  Vel_Omega : Subsystem
  Panel Velocities : Outport
  wires:
  Flexible defections/2(Del_v_flex) -> Sum/3
  Repmat function/1(Vrepmat) -> Sum/1
  Vel_Omega/1(Omegacrossr) -> Sum/2
  Flexible defections/1(Del_r_flex) -> Vel_Omega/2(Del_r_flex)
  Rigid States/1 -> Bus Selector/1
  Gain1/1 -> Vel_Omega/1(Omegab)
  Flexible States/1 -> Flexible defections/1(Flexible States)
  Bus Selector/2 -> Gain1/1  "<Omegab>"
  Bus Selector/1 -> Gain/1  "<Vb>"
  Gain/1 -> Repmat function/1(V)
  Sum/1 -> Panel Velocities/1

== system NL_Simulation/Force and Moment /Aerodynamic Model/Steady Aerodynamics/Total Wash/Flexible defections ==
  Flexible States : Inport
  Bus Selector1 : BusSelector  OutputSignals=EtaFlex,EtaFlexdot
  Phif_Translation : Constant  Value=AC.ModalStruc.Phif_aero_trans
  Product1 : Product  Multiplication=Matrix(*)
  Product2 : Product  Multiplication=Matrix(*)
  Reshape1 : Reshape  OutputDimensionality=Customize  OutputDimensions=[3,AC.Aero.NumPanels]
  Reshape2 : Reshape  OutputDimensionality=Customize  OutputDimensions=[3,AC.Aero.NumPanels]
  Del_r_flex : Outport
  Del_v_flex : Outport  Port=2
  wires:
  Product1/1 -> Reshape1/1
  Bus Selector1/2 -> Product2/2  "<EtaFlexdot>"
  Reshape1/1 -> Del_r_flex/1
  Flexible States/1 -> Bus Selector1/1
  Product2/1 -> Reshape2/1
  Phif_Translation/1 -> Product2/1, Product1/1
  Bus Selector1/1 -> Product1/2  "<EtaFlex>"
  Reshape2/1 -> Del_v_flex/1

== system NL_Simulation/Force and Moment /Aerodynamic Model/Steady Aerodynamics/Total Wash/Vel_Omega ==
  Omegab : Inport
  Del_r_flex : Inport  Port=2
  Cross Product Matrix : Tools_6dofSimulation/Cross Product Matrix  SystemSampleTime=-1
  Demux : Demux  Outputs=3
  Product : Product  Multiplication=Matrix(*)
  Sum : Sum
  rcg_colloc : Constant  Value=AC.Aero.VLMData.grid.r_cgcolloc
  Omegacrossr : Outport
  wires:
  Omegab/1 -> Demux/1
  Product/1 -> Omegacrossr/1
  Demux/2 -> Cross Product Matrix/2  "q"
  Demux/3 -> Cross Product Matrix/3  "r"
  Cross Product Matrix/1 -> Product/1
  Sum/1 -> Product/2
  Del_r_flex/1 -> Sum/1
  rcg_colloc/1 -> Sum/2
  Demux/1 -> Cross Product Matrix/1  "p"

== system NL_Simulation/Force and Moment /Aerodynamic Model/Steady Aerodynamics/Vortex Strength/Subsystem ==
  Flexible States : Inport
  "Ainv0 " : Constant  Value=AC.Aero.VLMData.Ainv0
  Bus Selector : BusSelector  OutputSignals=EtaFlex
  Subsystem : Subsystem
  Sum : Sum
  AIC : Outport
  wires:
  Sum/1 -> AIC/1  "AIC"
  "Ainv0 "/1 -> Sum/1
  Flexible States/1 -> Bus Selector/1
  Bus Selector/1 -> Subsystem/1(Eta_Flex)  "<EtaFlex>"
  Subsystem/1(AIC_Flex) -> Sum/2

== system NL_Simulation/Force and Moment /Aerodynamic Model/Unsteady Aerodynamics/Normal Forces/MACby2V ==
  Rigid States : Inport
  Bus Selector : BusSelector  OutputSignals=Vb
  Constant : Constant  Value=AC.Aero.MAC
  Gain : Gain  Gain=.5
  Product : Product  Inputs=*/
  Vs Calculation : Subsystem
  MACby2V : Outport
  wires:
  Vs Calculation/1(Vs) -> Product/2
  Rigid States/1 -> Bus Selector/1
  Product/1 -> MACby2V/1
  Bus Selector/1 -> Vs Calculation/1(<Vb>)  "<Vb>"
  Constant/1 -> Gain/1
  Gain/1 -> Product/1

== system NL_Simulation/Force and Moment /Aerodynamic Model/Unsteady Aerodynamics/Normal Forces/Subsystem1 ==
  Normal Wash Derivative : Inport
  b_over_V : Inport  Port=2
  B_lag : Gain  Gain=AC.Aero.DLMData.Blag  Multiplication=Matrix(K*u)
  Gain : Gain  Gain=AC.Aero.DLMData.Alag  Multiplication=Matrix(K*u)
  Lag : Integrator  InitialCondition=zeros(1776,1)
  Product : Product  Inputs=/*
  Sum : Sum  Inputs=|++
  Lag States : Outport
  wires:
  Normal Wash Derivative/1 -> B_lag/1
  B_lag/1 -> Sum/1
  Sum/1 -> Lag/1
  Lag/1 -> Product/2
  b_over_V/1 -> Product/1
  Product/1 -> Lag States/1, Gain/1
  Gain/1 -> Sum/2

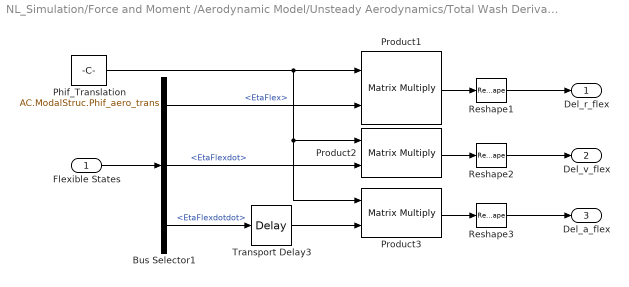
== system NL_Simulation/Force and Moment /Aerodynamic Model/Unsteady Aerodynamics/Total Wash Derivative/Flexible defections ==
  Flexible States : Inport
  Bus Selector1 : BusSelector  OutputSignals=EtaFlex,EtaFlexdot,EtaFlexdotdot
  Phif_Translation : Constant  Value=AC.ModalStruc.Phif_aero_trans
  Product1 : Product  Multiplication=Matrix(*)
  Product2 : Product  Multiplication=Matrix(*)
  Product3 : Product  Multiplication=Matrix(*)
  Reshape1 : Reshape  OutputDimensionality=Customize  OutputDimensions=[3,AC.Aero.NumPanels]
  Reshape2 : Reshape  OutputDimensionality=Customize  OutputDimensions=[3,AC.Aero.NumPanels]
  Reshape3 : Reshape  OutputDimensionality=Customize  OutputDimensions=[3,AC.Aero.NumPanels]
  Transport Delay3 : TransportDelay  DelayTime=0.001
  Del_r_flex : Outport
  Del_v_flex : Outport  Port=2
  Del_a_flex : Outport  Port=3
  wires:
  Product1/1 -> Reshape1/1
  Bus Selector1/2 -> Product2/2  "<EtaFlexdot>"
  Reshape1/1 -> Del_r_flex/1
  Flexible States/1 -> Bus Selector1/1
  Product2/1 -> Reshape2/1
  Bus Selector1/1 -> Product1/2  "<EtaFlex>"
  Reshape2/1 -> Del_v_flex/1
  Phif_Translation/1 -> Product3/1, Product2/1, Product1/1
  Bus Selector1/3 -> Transport Delay3/1  "<EtaFlexdotdot>"
  Product3/1 -> Reshape3/1
  Reshape3/1 -> Del_a_flex/1
  Transport Delay3/1 -> Product3/2

== system NL_Simulation/Force and Moment /Aerodynamic Model/Unsteady Aerodynamics/Total Wash Derivative/Vel_Omega ==
  Omegabdot : Inport
  Del_r_flex : Inport  Port=2
  Cross Product Matrix : Tools_6dofSimulation/Cross Product Matrix  SystemSampleTime=-1
  Demux : Demux  Outputs=3
  Product : Product  Multiplication=Matrix(*)
  Sum : Sum
  rcg_colloc : Constant  Value=AC.Aero.VLMData.grid.r_cgcolloc
  Omegacrossr : Outport
  wires:
  Omegabdot/1 -> Demux/1
  Product/1 -> Omegacrossr/1
  Demux/2 -> Cross Product Matrix/2  "q"
  Demux/3 -> Cross Product Matrix/3  "r"
  Cross Product Matrix/1 -> Product/1
  Sum/1 -> Product/2
  Del_r_flex/1 -> Sum/1
  rcg_colloc/1 -> Sum/2
  Demux/1 -> Cross Product Matrix/1  "p"

== system NL_Simulation/Force and Moment /Aerodynamic Model/Unsteady Aerodynamics/Total Wash Derivative/Vel_Omega1 ==
  Omegab : Inport
  Del_v_flex : Inport  Port=2
  Cross Product Matrix : Tools_6dofSimulation/Cross Product Matrix  SystemSampleTime=-1
  Demux : Demux  Outputs=3
  Product : Product  Multiplication=Matrix(*)
  Omegacrossr : Outport
  wires:
  Omegab/1 -> Demux/1
  Product/1 -> Omegacrossr/1
  Demux/2 -> Cross Product Matrix/2  "q"
  Demux/3 -> Cross Product Matrix/3  "r"
  Cross Product Matrix/1 -> Product/1
  Del_v_flex/1 -> Product/2
  Demux/1 -> Cross Product Matrix/1  "p"

== system NL_Simulation/Force and Moment /Aerodynamic Model/Steady Aerodynamics/Panel Forces Calculation/External Induced Velocity/Flexible defections ==
  Flexible States : Inport
  Bus Selector1 : BusSelector  OutputSignals=EtaFlex,EtaFlexdot
  Phif_Translation : Constant  Value=AC.ModalStruc.Phif_aero_trans
  Product1 : Product  Multiplication=Matrix(*)
  Product2 : Product  Multiplication=Matrix(*)
  Reshape1 : Reshape  OutputDimensionality=Customize  OutputDimensions=[3,AC.Aero.NumPanels]
  Reshape2 : Reshape  OutputDimensionality=Customize  OutputDimensions=[3,AC.Aero.NumPanels]
  Del_r_flex : Outport
  Del_v_flex : Outport  Port=2
  wires:
  Product1/1 -> Reshape1/1
  Bus Selector1/2 -> Product2/2  "<EtaFlexdot>"
  Reshape1/1 -> Del_r_flex/1
  Flexible States/1 -> Bus Selector1/1
  Product2/1 -> Reshape2/1
  Phif_Translation/1 -> Product2/1, Product1/1
  Bus Selector1/1 -> Product1/2  "<EtaFlex>"
  Reshape2/1 -> Del_v_flex/1

== system NL_Simulation/Force and Moment /Aerodynamic Model/Steady Aerodynamics/Panel Forces Calculation/External Induced Velocity/Vel_Omega ==
  Omegab : Inport
  Del_r_flex : Inport  Port=2
  Cross Product Matrix : Tools_6dofSimulation/Cross Product Matrix  SystemSampleTime=-1
  Demux : Demux  Outputs=3
  Product : Product  Multiplication=Matrix(*)
  Sum : Sum
  rcg_vortex : Constant  Value=AC.Aero.VLMData.grid.r_cgvortex
  Omegacrossr : Outport
  wires:
  Omegab/1 -> Demux/1
  Product/1 -> Omegacrossr/1
  Demux/2 -> Cross Product Matrix/2  "q"
  Demux/3 -> Cross Product Matrix/3  "r"
  Cross Product Matrix/1 -> Product/1
  Sum/1 -> Product/2
  Del_r_flex/1 -> Sum/1
  rcg_vortex/1 -> Sum/2
  Demux/1 -> Cross Product Matrix/1  "p"

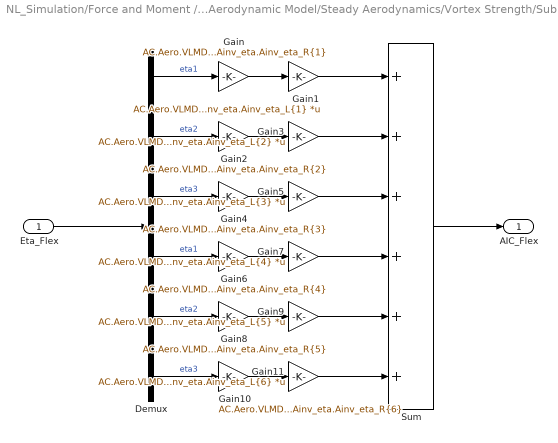
== system NL_Simulation/Force and Moment /Aerodynamic Model/Steady Aerodynamics/Vortex Strength/Subsystem/Subsystem ==
  Eta_Flex : Inport
  Demux : Demux  Outputs=6
  Gain : Gain  Gain=AC.Aero.VLMData.Ainv_eta.Ainv_eta_R{1}
  Gain1 : Gain  Gain=AC.Aero.VLMData.Ainv_eta.Ainv_eta_L{1}  Multiplication=Matrix(K*u)
  Gain10 : Gain  Gain=AC.Aero.VLMData.Ainv_eta.Ainv_eta_R{6}
  Gain11 : Gain  Gain=AC.Aero.VLMData.Ainv_eta.Ainv_eta_L{6}  Multiplication=Matrix(K*u)
  Gain2 : Gain  Gain=AC.Aero.VLMData.Ainv_eta.Ainv_eta_R{2}
  Gain3 : Gain  Gain=AC.Aero.VLMData.Ainv_eta.Ainv_eta_L{2}  Multiplication=Matrix(K*u)
  Gain4 : Gain  Gain=AC.Aero.VLMData.Ainv_eta.Ainv_eta_R{3}
  Gain5 : Gain  Gain=AC.Aero.VLMData.Ainv_eta.Ainv_eta_L{3}  Multiplication=Matrix(K*u)
  Gain6 : Gain  Gain=AC.Aero.VLMData.Ainv_eta.Ainv_eta_R{4}
  Gain7 : Gain  Gain=AC.Aero.VLMData.Ainv_eta.Ainv_eta_L{4}  Multiplication=Matrix(K*u)
  Gain8 : Gain  Gain=AC.Aero.VLMData.Ainv_eta.Ainv_eta_R{5}
  Gain9 : Gain  Gain=AC.Aero.VLMData.Ainv_eta.Ainv_eta_L{5}  Multiplication=Matrix(K*u)
  Sum : Sum  Inputs=++++++
  AIC_Flex : Outport
  wires:
  Gain2/1 -> Gain3/1
  Gain8/1 -> Gain9/1
  Gain11/1 -> Sum/6
  Gain3/1 -> Sum/2
  Demux/6 -> Gain10/1  "eta3"
  Gain1/1 -> Sum/1
  Gain/1 -> Gain1/1
  Gain5/1 -> Sum/3
  Demux/3 -> Gain4/1  "eta3"
  Gain7/1 -> Sum/4
  Gain9/1 -> Sum/5
  Demux/5 -> Gain8/1  "eta2"
  Gain4/1 -> Gain5/1
  Gain10/1 -> Gain11/1
  Demux/1 -> Gain/1  "eta1"
  Demux/2 -> Gain2/1  "eta2"
  Demux/4 -> Gain6/1  "eta1"
  Gain6/1 -> Gain7/1
  Sum/1 -> AIC_Flex/1
  Eta_Flex/1 -> Demux/1

== system NL_Simulation/Force and Moment /Aerodynamic Model/Unsteady Aerodynamics/Normal Forces/MACby2V/Vs Calculation ==
  <Vb> : Inport
  Demux : Demux  Outputs=3
  Product : Product
  Product1 : Product
  Product2 : Product
  Sqrt : Sqrt  SaturateOnIntegerOverflow=on
  Sum : Sum  Inputs=+++
  Vs : Outport
  wires:
  Sum/1 -> Sqrt/1
  Product/1 -> Sum/1
  Demux/3 -> Product2/1, Product2/2
  <Vb>/1 -> Demux/1
  Product1/1 -> Sum/2
  Demux/2 -> Product1/1, Product1/2
  Product2/1 -> Sum/3
  Sqrt/1 -> Vs/1
  Demux/1 -> Product/1, Product/2

== matlab function NL_Simulation/Force and Moment /Aerodynamic Model/Unsteady Aerodynamics/Total Wash Derivative/Repmat function ==
  data: Ab input; Abrepmat output; NumPanels parameter
function Abrepmat = fcn(Ab,NumPanels)
Abrepmat = repmat(Ab,1,NumPanels);
end

== matlab function NL_Simulation/Force and Moment /Aerodynamic Model/Steady Aerodynamics/Total Wash/Repmat function ==
  data: V input; Vrepmat output; NumPanels parameter
function Vrepmat = fcn(V,NumPanels)
Vrepmat = repmat(V,1,NumPanels);
end

== matlab function NL_Simulation/Force and Moment /Aerodynamic Model/Unsteady Aerodynamics/MATLAB Function ==
  data: nhat0 input; TotalForces output; NormalForces input
function TotalForces = fcn(nhat0,NormalForces)
%nhat0 = 3*888
%normalForce = 888*1
%TotalForce = 3*888;
Fx = zeros(888,1);
Fy = [zeros(552,1); NormalForces(553:888,1)];
Fz = [NormalForces(1:552,1); zeros(336,1)];

TotalForces = [Fx,Fy,Fz]'.*nhat0;

== matlab function NL_Simulation/Force and Moment /Aerodynamic Model/Steady Aerodynamics/N_hat/Axis-Angle to DCM/Replace Nhat ==
  data: Nhat1 input; Nhat1 output; NhatNew input; idx input
function Nhat1 = fcn(Nhat1,NhatNew,idx)
Nhat1(:,idx) = NhatNew;

== matlab function NL_Simulation/Force and Moment /Aerodynamic Model/Steady Aerodynamics/Panel Forces Calculation/External Induced Velocity/Repmat function ==
  data: V input; Vrepmat output; NumPanels parameter
function Vrepmat = fcn(V,NumPanels)
Vrepmat = repmat(V,1,NumPanels);
end

== matlab function NL_Simulation/Force and Moment /Aerodynamic Model/Steady Aerodynamics/Panel Forces Calculation/MATLAB Function ==
  data: V input; VcrossGammaLen output; Gamma_len input
function VcrossGammaLen = fcn(V,Gamma_len)
VcrossGammaLen = cross(V,Gamma_len,1);
end

== matlab function NL_Simulation/Force and Moment /Aerodynamic Model/Steady Aerodynamics/Panel Forces Calculation/Repmat function ==
  data: Gamma input; Gamma_rep output
function Gamma_rep = fcn(Gamma)
Gamma_rep = repmat(Gamma,1,3)';
end

== matlab function NL_Simulation/Force and Moment /Total Forces and Moments/MATLAB Function ==
  data: R input; SumRcrossF output; F input
function SumRcrossF = fcn(R,F)
SumRcrossF = sum(cross(R,F),2);
end
